simulink model "QUAD_With_IBS_Final"  (R2015a)
settings: Solver=ode45  StartTime=0.0  StopTime=10.0  RelTol=1e-3
libraries: simulink x10, commnoisgen2 x6
settings Model: Creator=Oussama  LastModifiedBy=Oussama

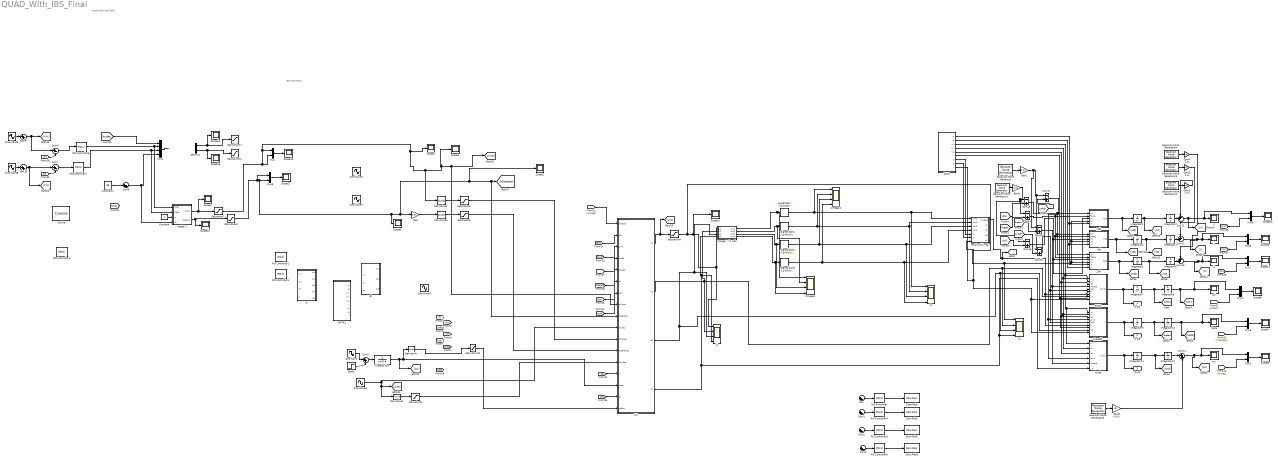
== system QUAD_With_IBS_Final ==
  note: IBS CONTROL
  note: used to extract data
  Bi : MATLAB Function  TreatAsAtomicUnit=on
  Constant : Constant
  Constant1 : Constant  Value=25
  Cosine : simulink/Lookup Tables/Cosine  Formula=cos(2*pi*u)  NumDataPoints=(2^5)+1  OutputWordLength=16  InternalRulePriority=Speed
  DATA : MATLAB Function  TreatAsAtomicUnit=on
  DATA1 : MATLAB Function  TreatAsAtomicUnit=on
  Demux1 : Demux  Outputs=2
  Derivative{,1..3} (4 alike) : Derivative
  Gain : Gain  Gain=0.01
  Gain1 : Gain  Gain=0.01
  Gain2 : Gain  Gain=0.03
  Gain3 : Gain  Gain=0.03
  Gain4 : Gain  Gain=0.03
  Gain5 : Gain  Gain=0.01
  Gain6 : Gain  Gain=0.0001
  Gaussian Noise Generator : commnoisgen2/Gaussian Noise Generator  m=0  d=1  s=41  Ts=0.02  frameBased=off  sampPerFrame=1  orient=off  outDataType=double
  Gaussian Noise Generator1 : commnoisgen2/Gaussian Noise Generator  m=0  d=1  s=41  Ts=0.02  frameBased=off  sampPerFrame=1  orient=off  outDataType=double
  Gaussian Noise Generator2 : commnoisgen2/Gaussian Noise Generator  m=0.3  d=1  s=41  Ts=5  frameBased=off  sampPerFrame=1  orient=off  outDataType=double
  Gaussian Noise Generator3 : commnoisgen2/Gaussian Noise Generator  m=0.3  d=1  s=41  Ts=12  frameBased=off  sampPerFrame=1  orient=off  outDataType=double
  Gaussian Noise Generator4 : commnoisgen2/Gaussian Noise Generator  m=0.3  d=1  s=41  Ts=7  frameBased=off  sampPerFrame=1  orient=off  outDataType=double
  Gaussian Noise Generator5 : commnoisgen2/Gaussian Noise Generator  m=0  d=1  s=41  Ts=0.02  frameBased=off  sampPerFrame=1  orient=off  outDataType=double
  Integrator{1..12} (12 alike) : Integrator
  Mux{,2..8} (8 alike) : Mux  Inputs=2
  Mux1 : Mux
  Omega i ^2  calc : MATLAB Function  TreatAsAtomicUnit=on
  Omegas : Scope  NumInputPorts=4
      settings: YMin=-5~-5~-5~-5  YMax=5~5~5~5  SaveName=ScopeData3
  PID Controller{,4..6} (4 alike) : simulink/Continuous/PID Controller  Controller=PID  TimeDomain=Continuous-time  SampleTime=-1  IntegratorMethod=Forward Euler  FilterMethod=Forward Euler  Form=Parallel  UseFilter=on  ControllerParametersSource=internal  P=0.696663945518539  I=69.3627675374527  D=0.000480635781112464  N=569.937710840054  InitialConditionSource=internal  InitialConditionForIntegrator=0  InitialConditionForFilter=0  ExternalReset=none  LimitOutput=off  UpperSaturationLimit=+12  LowerSaturationLimit=-12  LinearizeAsGain=on  AntiWindupMode=clamping  Kb=1  TrackingMode=off  Kt=1  PParamMin=[]  PParamMax=[]  IParamMin=[]  IParamMax=[]  DParamMin=[]  DParamMax=[]  NParamMin=[]  NParamMax=[]  KbParamMin=[]  KbParamMax=[]  KtParamMin=[]  KtParamMax=[]  POutMin=[]  POutMax=[]  IOutMin=[]  IOutMax=[]  DOutMin=[]  DOutMax=[]  NOutMin=[]  NOutMax=[]  KbOutMin=[]  KbOutMax=[]  KtOutMin=[]  KtOutMax=[]  IntegratorOutMin=[]  IntegratorOutMax=[]  FilterOutMin=[]  FilterOutMax=[]  SumOutMin=[]  SumOutMax=[]  SumI1OutMin=[]  SumI1OutMax=[]  SumI2OutMin=[]  SumI2OutMax=[]  SumI3OutMin=[]  SumI3OutMax=[]  SumDOutMin=[]  SumDOutMax=[]  SaturationOutMin=[]  SaturationOutMax=[]  IntegratorContinuousStateAttributes=''  IntegratorStateMustResolveToSignalObject=off  IntegratorRTWStateStorageClass=Auto  FilterContinuousStateAttributes=''  FilterStateMustResolveToSignalObject=off  FilterRTWStateStorageClass=Auto  DifferentiatorICPrevScaledInput=0  DifferentiatorOutMin=[]  DifferentiatorOutMax=[]
  PID Controller1 : simulink/Continuous/PID Controller  Controller=PID  TimeDomain=Continuous-time  SampleTime=-1  IntegratorMethod=Forward Euler  FilterMethod=Forward Euler  Form=Parallel  UseFilter=on  ControllerParametersSource=internal  P=0.8  I=0.4  D=2  N=100  InitialConditionSource=internal  InitialConditionForIntegrator=0  InitialConditionForFilter=0  ExternalReset=none  LimitOutput=off  UpperSaturationLimit=inf  LowerSaturationLimit=-inf  LinearizeAsGain=on  AntiWindupMode=none  Kb=1  TrackingMode=off  Kt=1  PParamMin=[]  PParamMax=[]  IParamMin=[]  IParamMax=[]  DParamMin=[]  DParamMax=[]  NParamMin=[]  NParamMax=[]  KbParamMin=[]  KbParamMax=[]  KtParamMin=[]  KtParamMax=[]  POutMin=[]  POutMax=[]  IOutMin=[]  IOutMax=[]  DOutMin=[]  DOutMax=[]  NOutMin=[]  NOutMax=[]  KbOutMin=[]  KbOutMax=[]  KtOutMin=[]  KtOutMax=[]  IntegratorOutMin=[]  IntegratorOutMax=[]  FilterOutMin=[]  FilterOutMax=[]  SumOutMin=[]  SumOutMax=[]  SumI1OutMin=[]  SumI1OutMax=[]  SumI2OutMin=[]  SumI2OutMax=[]  SumI3OutMin=[]  SumI3OutMax=[]  SumDOutMin=[]  SumDOutMax=[]  SaturationOutMin=[]  SaturationOutMax=[]  IntegratorContinuousStateAttributes=''  IntegratorStateMustResolveToSignalObject=off  IntegratorRTWStateStorageClass=Auto  FilterContinuousStateAttributes=''  FilterStateMustResolveToSignalObject=off  FilterRTWStateStorageClass=Auto  DifferentiatorICPrevScaledInput=0  DifferentiatorOutMin=[]  DifferentiatorOutMax=[]
  PID Controller2 : simulink/Continuous/PID Controller  Controller=PID  TimeDomain=Continuous-time  SampleTime=-1  IntegratorMethod=Forward Euler  FilterMethod=Forward Euler  Form=Parallel  UseFilter=on  ControllerParametersSource=internal  P=1.1  I=0.5  D=4  N=100  InitialConditionSource=internal  InitialConditionForIntegrator=0  InitialConditionForFilter=0  ExternalReset=none  LimitOutput=off  UpperSaturationLimit=inf  LowerSaturationLimit=-inf  LinearizeAsGain=on  AntiWindupMode=none  Kb=1  TrackingMode=off  Kt=1  PParamMin=[]  PParamMax=[]  IParamMin=[]  IParamMax=[]  DParamMin=[]  DParamMax=[]  NParamMin=[]  NParamMax=[]  KbParamMin=[]  KbParamMax=[]  KtParamMin=[]  KtParamMax=[]  POutMin=[]  POutMax=[]  IOutMin=[]  IOutMax=[]  DOutMin=[]  DOutMax=[]  NOutMin=[]  NOutMax=[]  KbOutMin=[]  KbOutMax=[]  KtOutMin=[]  KtOutMax=[]  IntegratorOutMin=[]  IntegratorOutMax=[]  FilterOutMin=[]  FilterOutMax=[]  SumOutMin=[]  SumOutMax=[]  SumI1OutMin=[]  SumI1OutMax=[]  SumI2OutMin=[]  SumI2OutMax=[]  SumI3OutMin=[]  SumI3OutMax=[]  SumDOutMin=[]  SumDOutMax=[]  SaturationOutMin=[]  SaturationOutMax=[]  IntegratorContinuousStateAttributes=''  IntegratorStateMustResolveToSignalObject=off  IntegratorRTWStateStorageClass=Auto  FilterContinuousStateAttributes=''  FilterStateMustResolveToSignalObject=off  FilterRTWStateStorageClass=Auto  DifferentiatorICPrevScaledInput=0  DifferentiatorOutMin=[]  DifferentiatorOutMax=[]
  PID Controller3 : simulink/Continuous/PID Controller  Controller=PID  TimeDomain=Continuous-time  SampleTime=-1  IntegratorMethod=Forward Euler  FilterMethod=Forward Euler  Form=Parallel  UseFilter=on  ControllerParametersSource=internal  P=3  I=0.5  D=0.9  N=100  InitialConditionSource=internal  InitialConditionForIntegrator=0  InitialConditionForFilter=0  ExternalReset=none  LimitOutput=off  UpperSaturationLimit=inf  LowerSaturationLimit=-inf  LinearizeAsGain=on  AntiWindupMode=none  Kb=1  TrackingMode=off  Kt=1  PParamMin=[]  PParamMax=[]  IParamMin=[]  IParamMax=[]  DParamMin=[]  DParamMax=[]  NParamMin=[]  NParamMax=[]  KbParamMin=[]  KbParamMax=[]  KtParamMin=[]  KtParamMax=[]  POutMin=[]  POutMax=[]  IOutMin=[]  IOutMax=[]  DOutMin=[]  DOutMax=[]  NOutMin=[]  NOutMax=[]  KbOutMin=[]  KbOutMax=[]  KtOutMin=[]  KtOutMax=[]  IntegratorOutMin=[]  IntegratorOutMax=[]  FilterOutMin=[]  FilterOutMax=[]  SumOutMin=[]  SumOutMax=[]  SumI1OutMin=[]  SumI1OutMax=[]  SumI2OutMin=[]  SumI2OutMax=[]  SumI3OutMin=[]  SumI3OutMax=[]  SumDOutMin=[]  SumDOutMax=[]  SaturationOutMin=[]  SaturationOutMax=[]  IntegratorContinuousStateAttributes=''  IntegratorStateMustResolveToSignalObject=off  IntegratorRTWStateStorageClass=Auto  FilterContinuousStateAttributes=''  FilterStateMustResolveToSignalObject=off  FilterRTWStateStorageClass=Auto  DifferentiatorICPrevScaledInput=0  DifferentiatorOutMin=[]  DifferentiatorOutMax=[]
  PID Controller7 : simulink/Continuous/PID Controller  Controller=PID  TimeDomain=Continuous-time  SampleTime=-1  IntegratorMethod=Forward Euler  FilterMethod=Forward Euler  Form=Parallel  UseFilter=on  ControllerParametersSource=internal  P=1.9  I=2.5  D=10  N=100  InitialConditionSource=internal  InitialConditionForIntegrator=0  InitialConditionForFilter=0  ExternalReset=none  LimitOutput=off  UpperSaturationLimit=inf  LowerSaturationLimit=-inf  LinearizeAsGain=on  AntiWindupMode=none  Kb=1  TrackingMode=off  Kt=1  PParamMin=[]  PParamMax=[]  IParamMin=[]  IParamMax=[]  DParamMin=[]  DParamMax=[]  NParamMin=[]  NParamMax=[]  KbParamMin=[]  KbParamMax=[]  KtParamMin=[]  KtParamMax=[]  POutMin=[]  POutMax=[]  IOutMin=[]  IOutMax=[]  DOutMin=[]  DOutMax=[]  NOutMin=[]  NOutMax=[]  KbOutMin=[]  KbOutMax=[]  KtOutMin=[]  KtOutMax=[]  IntegratorOutMin=[]  IntegratorOutMax=[]  FilterOutMin=[]  FilterOutMax=[]  SumOutMin=[]  SumOutMax=[]  SumI1OutMin=[]  SumI1OutMax=[]  SumI2OutMin=[]  SumI2OutMax=[]  SumI3OutMin=[]  SumI3OutMax=[]  SumDOutMin=[]  SumDOutMax=[]  SaturationOutMin=[]  SaturationOutMax=[]  IntegratorContinuousStateAttributes=''  IntegratorStateMustResolveToSignalObject=off  IntegratorRTWStateStorageClass=Auto  FilterContinuousStateAttributes=''  FilterStateMustResolveToSignalObject=off  FilterRTWStateStorageClass=Auto  DifferentiatorICPrevScaledInput=0  DifferentiatorOutMin=[]  DifferentiatorOutMax=[]
  PID Controller8 : simulink/Continuous/PID Controller  Controller=PID  TimeDomain=Continuous-time  SampleTime=-1  IntegratorMethod=Forward Euler  FilterMethod=Forward Euler  Form=Parallel  UseFilter=on  ControllerParametersSource=internal  P=2  I=2  D=8  N=100  InitialConditionSource=internal  InitialConditionForIntegrator=0  InitialConditionForFilter=0  ExternalReset=none  LimitOutput=off  UpperSaturationLimit=inf  LowerSaturationLimit=-inf  LinearizeAsGain=on  AntiWindupMode=none  Kb=1  TrackingMode=off  Kt=1  PParamMin=[]  PParamMax=[]  IParamMin=[]  IParamMax=[]  DParamMin=[]  DParamMax=[]  NParamMin=[]  NParamMax=[]  KbParamMin=[]  KbParamMax=[]  KtParamMin=[]  KtParamMax=[]  POutMin=[]  POutMax=[]  IOutMin=[]  IOutMax=[]  DOutMin=[]  DOutMax=[]  NOutMin=[]  NOutMax=[]  KbOutMin=[]  KbOutMax=[]  KtOutMin=[]  KtOutMax=[]  IntegratorOutMin=[]  IntegratorOutMax=[]  FilterOutMin=[]  FilterOutMax=[]  SumOutMin=[]  SumOutMax=[]  SumI1OutMin=[]  SumI1OutMax=[]  SumI2OutMin=[]  SumI2OutMax=[]  SumI3OutMin=[]  SumI3OutMax=[]  SumDOutMin=[]  SumDOutMax=[]  SaturationOutMin=[]  SaturationOutMax=[]  IntegratorContinuousStateAttributes=''  IntegratorStateMustResolveToSignalObject=off  IntegratorRTWStateStorageClass=Auto  FilterContinuousStateAttributes=''  FilterStateMustResolveToSignalObject=off  FilterRTWStateStorageClass=Auto  DifferentiatorICPrevScaledInput=0  DifferentiatorOutMin=[]  DifferentiatorOutMax=[]
  Phidd : MATLAB Function  TreatAsAtomicUnit=on
  Saturation10 : Saturate  UpperLimit=50  LowerLimit=-50
  Saturation11 : Saturate  UpperLimit=0.4  LowerLimit=-0.4
  Saturation12 : Saturate  UpperLimit=0.4  LowerLimit=-0.4
  Saturation4 : Saturate  UpperLimit=25  LowerLimit=1
  Saturation5 : Saturate  UpperLimit=50  LowerLimit=-50
  Saturation6 : Saturate  UpperLimit=50  LowerLimit=-50
  Saturation7 : Saturate  UpperLimit=0.35  LowerLimit=-0.35
  Saturation8 : Saturate  UpperLimit=0.35  LowerLimit=-0.35
  Saturation9 : Saturate  UpperLimit=pi  LowerLimit=-pi
  Scope{1..17} (17 alike) : Scope
      Scope1 settings: TimeRange=10  YMin=-0.504  YMax=-0.491
      Scope10 settings: YMin=4  YMax=5.75  SaveName=xdata
      Scope11 settings: YMin=7.955  YMax=7.9725  SaveName=zdata
      Scope12 settings: YMin=1.5708  YMax=1.5708
      Scope13 settings: TimeRange=10  YMin=-0.504  YMax=-0.491  SaveName=ScopeData17
      Scope14 settings: SaveName=ScopeData18
      Scope15 settings: TimeRange=10  YMin=-1.53062  YMax=-1.53062  SaveName=ScopeData19
      Scope16 settings: YMin=0.399992  YMax=0.400001  SaveName=ScopeData20
      Scope17 settings: TimeRange=10  YMin=-0.2  YMax=-0.185  SaveName=ScopeData21
      Scope2 settings: SaveName=ScopeData8
      Scope3 settings: SaveName=ScopeData9
      Scope4 settings: TimeRange=10  YMin=-0.504  YMax=-0.491  SaveName=ScopeData10
      Scope5 settings: YMin=1.49226  YMax=1.64934  SaveName=ScopeData11
      Scope6 settings: YMin=-0.125  YMax=0.125  SaveName=phi_ang
      Scope7 settings: YMin=-0.525  YMax=-0.275  SaveName=theta_ang
      Scope8 settings: YMin=-0.002  YMax=0  SaveName=ksi_ang
      Scope9 settings: YMin=-15  YMax=7.5  SaveName=ydata
  Signed Sqrt{,1..3} (4 alike) : Sqrt  Operator=signedSqrt  SaturateOnIntegerOverflow=on
  Sine Wave : Sin  Amplitude=0  Frequency=0.5  SampleTime=0
  Sine Wave2 : Sin  Amplitude=0.3  Frequency=0.6  SampleTime=0
  Sine Wave4 : Sin  Amplitude=0.2  Frequency=0.3  SampleTime=0
  Sine Wave5 : Sin  Amplitude=0  Frequency=0.3  SampleTime=0
  Sine Wave7 : Sin  Amplitude=0.3  Frequency=0.6  SampleTime=0
  Sine Wave8 : Sin  Amplitude=10  Frequency=4*0.06  SampleTime=0
  Sine Wave9 : Sin  Amplitude=5  Frequency=5*0.06  Phase=3.14/2  SampleTime=0
  Step1 : Step  After=5  SampleTime=0
  Sum{,1..3,7,9} (6 alike) : Sum  Inputs=|+-
  Sum{5..6,8,10,14} (5 alike) : Sum  Inputs=|++
  Sum11 : Sum  Inputs=++|
  Sum12 : Sum  Inputs=++|
  Sum13 : Sum  Inputs=++|
  Sum{4,15..19} (6 alike) : Sum  Inputs=-+
  Transfer Fcn : TransferFcn  Denominator=[1 0.4]
  Ui : Scope  NumInputPorts=4
      settings: YMin=-5~-5~-5~-5  YMax=5~5~5~5  SaveName=ScopeData15
  Uiii : MATLAB Function  TreatAsAtomicUnit=on
  X : Scope
      settings: YMin=3.81  YMax=3.95  SaveName=ScopeData6
  X1 : Scope  NumInputPorts=4
      settings: YMin=-5~-5~-5~-5  YMax=5~5~5~5  SaveName=ScopeData16
  X2 : Scope  NumInputPorts=4
      settings: YMin=-5~-5~-5~-5  YMax=5~5~5~5  SaveName=ScopeData7
  Xdd : MATLAB Function  TreatAsAtomicUnit=on
  Y : Scope
      settings: YMin=-0.01095  YMax=-0.0103  SaveName=ScopeData5
  Ydd : MATLAB Function  TreatAsAtomicUnit=on
  "Z " : Scope
      settings: YMin=7.615  YMax=7.6215  SaveName=ScopeData2
  Zdd : MATLAB Function  TreatAsAtomicUnit=on
  Zero-Pole{,1..3} (4 alike) : ZeroPole  Zeros=[]  Poles=[-22.5]  Gain=[509]
  "ai " : MATLAB Function  TreatAsAtomicUnit=on
  angles 1 : MATLAB Function  TreatAsAtomicUnit=on
  ksi : Scope
      settings: SaveName=ksiangle
  ksidd : MATLAB Function  TreatAsAtomicUnit=on
  omegas2 : Scope  NumInputPorts=4
      settings: YMin=-5~-5~-5~-5  YMax=5~5~5~5  SaveName=ScopeData4
  phi : Scope
      settings: SaveName=phiangle
  recalc of Ui real : MATLAB Function  TreatAsAtomicUnit=on
  theta : Scope
      settings: SaveName=thetaangle
  thetadd : MATLAB Function  TreatAsAtomicUnit=on
  Out2 : Outport
  Out3 : Outport  Port=2
  Out4 : Outport  Port=3
  wires:
  Xdd/1(Xdd) -> [Xdd], Integrator1/1
  Ydd/1(Ydd) -> [Ydd], Integrator3/1
  Zdd/1(Zdd) -> [zdd], Integrator5/1
  Phidd/1(phidd) -> Out2/1, Integrator7/1
  Integrator7/1 -> [phid], Integrator8/1
  thetadd/1(thetadd) -> Out3/1, Integrator9/1
  Integrator9/1 -> [thetad], Integrator10/1
  ksidd/1(ksidd) -> Out4/1, Integrator11/1
  Integrator11/1 -> [ksid], Integrator12/1
  Integrator8/1 -> Mux2/1, phi/1, [phi]
  DATA/1(m) -> Zdd/5(m), Ydd/5(m), Xdd/5(m)
  DATA/2(g) -> Zdd/6(g)
  DATA/3(Ixx) -> ksidd/1(Ixx), thetadd/1(Ixx), Phidd/1(Ixx)
  DATA/4(Iyy) -> Phidd/2(Iyy), ksidd/2(Iyy), thetadd/2(Iyy)
  DATA/5(Izz) -> thetadd/3(Izz), ksidd/3(Izz), Phidd/3(Izz)
  DATA/6(J) -> thetadd/7(J), Phidd/7(J)
  Sum15/1 -> Zdd/1(phi), Ydd/1(phi), Xdd/1(phi)
  Sum4/1 -> Zdd/2(theta), Ydd/2(theta), Xdd/2(theta)
  Sum16/1 -> Xdd/3(ksi), Zdd/3(ksi), Ydd/3(ksi)
  Sum18/1 -> Phidd/4(thetad), ksidd/5(thetad)
  Sum19/1 -> Phidd/5(ksid), thetadd/5(ksid)
  Sum17/1 -> ksidd/4(phid), thetadd/4(phid)
  recalc of Ui real/1(omega) -> [omega], thetadd/6(omega), Phidd/6(omega)
  DATA/7(b) -> recalc of Ui real/5(b)
  DATA/8(d) -> recalc of Ui real/6(d)
  Uiii/4(U4) -> ksidd/6(u4), X2/4, Ui/4, Omega i ^2  calc/4(u4)
  Uiii/3(U3) -> X2/3, thetadd/8(u3), Ui/3, Omega i ^2  calc/3(u3)
  Uiii/2(U2) -> X2/2, Phidd/8(u2), Omega i ^2  calc/2(u2), Ui/2
  Omega i ^2  calc/1(om1) -> Omegas/1, Signed Sqrt/1
  Omega i ^2  calc/2(om2) -> Omegas/2, Signed Sqrt1/1
  Omega i ^2  calc/3(om3) -> Omegas/3, Signed Sqrt2/1
  Omega i ^2  calc/4(om4) -> Omegas/4, Signed Sqrt3/1
  Gain5/1 -> Sum16/1, Sum4/1, Sum15/1
  [phi] -> Sum15/2
  [theta] -> Sum4/2
  [ksi] -> Sum16/2
  Gain1/1 -> Sum18/1, Sum19/1, Sum17/1
  [phid] -> Sum17/2
  [thetad] -> Sum18/2
  [ksid] -> Sum19/2
  Saturation4/1 -> X2/1, Zdd/4(u1), Ydd/4(u1), Xdd/4(u1), Scope14/1, Ui/1, Omega i ^2  calc/1(u1)
  Integrator5/1 -> [zd], Integrator6/1
  Integrator3/1 -> [Yd], Integrator4/1
  Integrator1/1 -> [Xd], Integrator2/1
  DATA/9(l) -> Phidd/9(l), thetadd/9(l), recalc of Ui real/7(l)
  [phides] -> Mux2/2
  Mux2/1 -> Scope6/1
  Integrator10/1 -> [theta], Mux3/1, theta/1
  [thetades] -> Mux3/2
  Mux3/1 -> Scope7/1
  Sum14/1 -> [ksi], Mux4/1, ksi/1
  [ksides] -> Mux4/2
  Mux4/1 -> Scope8/1
  Sum12/1 -> [Y], Mux5/1, Y/1
  [YYY] -> Mux5/2
  Mux5/1 -> Scope9/1
  Sum11/1 -> [X], Mux6/1, X/1
  [XXX] -> Mux6/2
  Mux6/1 -> Scope10/1
  Sum13/1 -> Mux7/1, "Z "/1, [Z]
  [zzz] -> Mux7/2
  Mux7/1 -> Scope11/1
  Sum5/1 -> Transfer Fcn/1
  Derivative/1 -> Saturation10/1
  Sine Wave5/1 -> Derivative1/1, [ksides], Uiii/10(ksides)
  Derivative1/1 -> Saturation9/1
  [omega] -> Uiii/1(omega)
  Uiii/1(U1) -> [U11], Saturation4/1
  Step1/1 -> Sum5/2
  Sine Wave/1 -> Sum5/1
  Derivative2/1 -> Saturation5/1
  Derivative3/1 -> Saturation6/1
  ? -> Sum/2
  Sum/1 -> PID Controller/1
  PID Controller/1 -> Zero-Pole/1
  ? -> Sum1/2
  Sum1/1 -> PID Controller4/1
  PID Controller4/1 -> Zero-Pole1/1
  ? -> Sum2/2
  Sum2/1 -> PID Controller5/1
  PID Controller5/1 -> Zero-Pole2/1
  ? -> Sum3/2
  Sum3/1 -> PID Controller6/1
  PID Controller6/1 -> Zero-Pole3/1
  Signed Sqrt/1 -> X1/1, recalc of Ui real/1(om1), omegas2/1
  Signed Sqrt1/1 -> X1/2, recalc of Ui real/2(om2), omegas2/2
  Signed Sqrt2/1 -> X1/3, recalc of Ui real/3(om3), omegas2/3
  Signed Sqrt3/1 -> X1/4, recalc of Ui real/4(om4), omegas2/4
  [phi] -> Uiii/2(phi)
  [theta] -> Uiii/4(theta)
  [thetad] -> Uiii/5(thetad)
  [ksi] -> Uiii/6(ksi)
  [ksid] -> Uiii/7(ksid)
  [phid] -> Uiii/3(phid)
  Saturation9/1 -> Uiii/13(ksiddes)
  Saturation7/1 -> Mux/2, Derivative2/1, Uiii/8(phides), [phides], Scope3/1, Scope4/1, Mux/1
  Saturation8/1 -> Mux8/2, Scope5/1, Gain/1, Scope2/1, Uiii/9(thetades), [thetades], Mux8/1
  Saturation5/1 -> Uiii/11(phiddes)
  Saturation6/1 -> Uiii/12(thetaddes)
  [Z] -> Uiii/14(z)
  [zd] -> Uiii/16(zd)
  Saturation10/1 -> Uiii/17(zddes)
  Mux1/1 -> ?
  Demux1/1 -> Scope15/1, Saturation11/1
  Demux1/2 -> Saturation12/1, Scope16/1
  ? -> Demux1/1
  [ksides] -> Mux1/1
  Sum6/1 -> Mux1/4, angles 1/4(U1)
  Constant/1 -> angles 1/3(m)
  angles 1/1(phitrk) -> Saturation7/1, Scope1/1
  angles 1/2(thetatrk) -> Scope12/1, Saturation8/1
  Mux/1 -> Scope13/1
  Mux8/1 -> Scope17/1
  Sum8/1 -> Sum9/1, [XXX]
  Sum10/1 -> [YYY], Sum7/1
  Sine Wave8/1 -> Sum10/1
  Sine Wave9/1 -> Sum8/1
  Sum9/1 -> PID Controller8/1
  Sum7/1 -> PID Controller7/1
  [X] -> Sum9/2
  [Y] -> Sum7/2
  Constant1/1 -> Sum6/1
  PID Controller7/1 -> angles 1/2(Ydes), Mux1/3
  PID Controller8/1 -> angles 1/1(Xdes), Mux1/2
  Gain/1 -> Derivative3/1
  Transfer Fcn/1 -> [zzz], Uiii/15(zdes), Derivative/1
  Gaussian Noise Generator2/1 -> Gain2/1
  Gain2/1 -> Sum11/1
  Gaussian Noise Generator3/1 -> Gain3/1
  Gain3/1 -> Sum12/1
  Gaussian Noise Generator4/1 -> Gain4/1
  Gain4/1 -> Sum13/1
  Gaussian Noise Generator/1 -> Gain1/1
  Gaussian Noise Generator1/1 -> Gain5/1
  Integrator2/1 -> Sum11/2
  Integrator4/1 -> Sum12/2
  Integrator6/1 -> Sum13/2
  Gaussian Noise Generator5/1 -> Gain6/1
  Integrator12/1 -> Sum14/1
  Gain6/1 -> Sum14/2

== matlab function QUAD_With_IBS_Final/Ydd ==
  data: phi input; Ydd output; theta input; ksi input; u1 input; m input
function Ydd = fcn(phi,theta, ksi,u1,m)
m=1;

Ydd=(-cos(ksi)*sin(phi)+sin(ksi)*sin(theta)*cos(phi))*u1/m;

== matlab function QUAD_With_IBS_Final/Zdd ==
  data: phi input; Zdd output; theta input; ksi input; u1 input; m input; g input
function Zdd = fcn(phi,theta, ksi,u1,m,g)
m=1;
g=9.81;

Zdd=-g+(cos(theta)*cos(phi))*u1/m;

== matlab function QUAD_With_IBS_Final/DATA ==
  data: m output; g output; Ixx output; Iyy output; Izz output; J output; b output; d output; l output
function [m,g,Ixx,Iyy,Izz,J,b,d,l] = fcn
m=1;
g=9.81;

Ixx=1*0.008;
Iyy=1*0.008;
Izz=1*0.015;
b=0.0001;
d=0.000001;
l=0.25;
J=0.0001;

== matlab function QUAD_With_IBS_Final/Phidd ==
  data: Ixx input; Iyy input; phidd output; Izz input; thetad input; ksid input; omega input; J input; u2 input; l input
function phidd = fcn(Ixx,Iyy,Izz,thetad, ksid,omega,J,u2,l)


phidd=1/Ixx*((Iyy-Izz)*thetad*ksid-J*thetad*omega+l*u2);

== matlab function QUAD_With_IBS_Final/thetadd ==
  data: Ixx input; Iyy input; thetadd output; Izz input; phid input; ksid input; omega input; J input; u3 input; l input
function thetadd = fcn(Ixx,Iyy,Izz,phid, ksid,omega,J,u3,l)


thetadd=1/Iyy*((Izz-Ixx)*phid*ksid+J*phid*omega+l*u3);

== matlab function QUAD_With_IBS_Final/ksidd ==
  data: Ixx input; Iyy input; ksidd output; Izz input; phid input; thetad input; u4 input
function ksidd = fcn(Ixx,Iyy,Izz,phid, thetad,u4)


ksidd=1/Izz*((Ixx-Iyy)*phid*thetad+u4);

== matlab function QUAD_With_IBS_Final/Omega i ^2  calc ==
  data: u1 input; om1 output; u2 input; u3 input; u4 input; om2 output; om3 output; om4 output
function [om1,om2,om3,om4] = fcn(u1,u2,u3,u4)
%#codegen
b=0.0001;
d=0.000001;
l=0.25;
A=[ 1/(4*b),0, -1/(2*b*l), -1/(4*d);1/(4*b), -1/(2*b*l),0,  1/(4*d); 1/(4*b),  0,  1/(2*b*l), -1/(4*d);1/(4*b),1/(2*b*l), 0,  1/(4*d)];
B=A*[u1;u2;u3;u4];
%[om1;om2;om3;om4]
om1= B(1);
om2=B(2);
om3=B(3);
om4=B(4);

== matlab function QUAD_With_IBS_Final/ai  ==
  data: Ixx input; a1 output; Iyy input; Izz input; a2 output; a3 output; a4 output; a5 output; Jr input
function [a1,a2,a3,a4,a5] = fcn(Ixx,Iyy,Izz,Jr)
a1=(Iyy-Izz)/Ixx;
a2=-Jr/Ixx;
a3=(Izz-Ixx)/Iyy;
a4=Jr/Iyy;
a5=(Ixx-Iyy)/Izz;

== matlab function QUAD_With_IBS_Final/Xdd ==
  data: phi input; Xdd output; theta input; ksi input; u1 input; m input
function Xdd = fcn(phi,theta, ksi,u1,m)


Xdd=(sin(ksi)*sin(phi)+cos(ksi)*sin(theta)*cos(phi))*u1/m;

== matlab function QUAD_With_IBS_Final/recalc of Ui real ==
  data: om1 input; omega output; om2 input; om3 input; om4 input; b input; d input; l input; u1 output; u2 output; u3 output; u4 output
function [omega, u1,u2,u3,u4] = fcn(om1,om2,om3,om4,b,d,l)

l=l;
omega=-om1+om2-om3+om4;
u1=b*(om1^2+om2^2+om3^2+om4^2);
u2=b*(om4^2-om2^2);
u3=b*(om3^2-om1^2);
u4=d*(om4^2+om2^2-om1^2-om3^2);

== matlab function QUAD_With_IBS_Final/Bi ==
  data: l input; Ixx input; b1 output; Iyy input; Izz input; b2 output; b3 output
function [b1,b2,b3] = fcn(l,Ixx,Iyy,Izz)

b1= l/Ixx;
b2= l/Iyy;
b3= l/Izz;

== matlab function QUAD_With_IBS_Final/angles 1 ==
  data: Xdes input; phitrk output; Ydes input; m input; U1 input; thetatrk output
function [phitrk,thetatrk]  = fcn(Xdes,Ydes, m,U1)
%#codegen
if U1<=5
    phitrk=0;
else
    if (abs(Ydes*m/U1) >= 0.3)
        phitrk= -sign(Ydes*m/U1)*pi/10;
    else
    phitrk=-asin(Ydes*m/U1);
    end
end
%%%%%%%%%%%%%%%%%%
if U1<=5
    thetatrk=0;
elseif (abs( Xdes*m/(U1*cos(phitrk)) ) >= 0.3 )
        thetatrk = sign( Xdes*m/(U1*cos(phitrk)) )*pi/10 ;
    else
    thetatrk=asin(Xdes*m/(U1*cos(phitrk)) );
end

    
%%%%%%%%%%%%
if phitrk > pi/3
    phitrk=pi/3;
end
if phitrk < -pi/3
    phitrk=-pi/3;
end
%%%%%%%%%%%%%%%
if thetatrk > pi/3
    thetatrk=pi/3;
end
if thetatrk < -pi/3
    thetatrk=-pi/3;
end

== matlab function QUAD_With_IBS_Final/DATA1 ==
  data: m output; g output; Ixx output; Iyy output; Izz output; J output; b output; d output; l output
function [m,g,Ixx,Iyy,Izz,J,b,d,l] = fcn
m=1;
g=9.81;

Ixx=1*0.008;
Iyy=1*0.008;
Izz=1*0.015;
b=0.0001;
d=0.000001;
l=0.25;
J=0.0001;

== matlab function QUAD_With_IBS_Final/Uiii ==
  data: omega input; phi input; phid input; theta input; thetad input; ksi input; ksid input; phides input; U1 output; U2 output; thetades input; ksides input; phiddes input; thetaddes input; ksiddes input; U3 output; U4 output; z input; zdes input; zd input; zddes input
function [U1,U2,U3,U4] = fcn(omega,phi,phid,theta,thetad,ksi,ksid,phides,thetades,ksides,phiddes,thetaddes,ksiddes,z,zdes,zd,zddes)
%%%%%%%%%%%%%%%%%%%%%%%%%%%%%%%%%%%%%%%%%%%%%%%%%%%%%%%%%%%%%
%%%%%%%%%%%%%%%%%%%%%%%%%%%%%%%%%%%%%%%%%%%%%%%%%%%%%%%%%%%%%

m=1;
g=9.81;

Ixx=1*0.008;
Iyy=1*0.008;
Izz=1*0.015;
b=0.0001;
d=0.000001;
l=0.25;
J=0.0001;
%%%%%%%%%%%%%%%%%%%%%%%%%%%%%%%%%%%%%%%%%%%%%%%%%%%%%%%%%%%%%
%%%%%%%%%%%%%%%%%%%%%%%%%%%%%%%%%%%%%%%%%%%%%%%%%%%%%%%%%%%%%

a1=(Iyy-Izz)/Ixx;
a2=-J/Ixx;
a3=(Izz-Ixx)/Iyy;
a4=J/Iyy;
a5=(Ixx-Iyy)/Izz;
%%%%%%%%%%%%%%%%%%%%%%%%%%%%%%%%%%%%%%%%%%%%%%%%%%%%%%%%%%%%%
%%%%%%%%%%%%%%%%%%%%%%%%%%%%%%%%%%%%%%%%%%%%%%%%%%%%%%%%%%%%%
b1= l/Ixx;
b2= l/Iyy;
b3= l/Izz;

%%%%%%%%%%%%%%%%%%%%%%%%%%%%%%%%%%%%%%%%%%%%%%%%%%%%%%%%%%%%%
%%%%%%%%%%%%%%%%%%%%%%%%%%%%%%%%%%%%%%%%%%%%%%%%%%%%%%%%%%%%%

k1=5.3;
k2=2.9;
k3=4.4;
k4=3.7;
k5=3.5;
k6=2.6;
k7=4.7;
k8=2.8;

% k7=1.7;
% k8=0.8;
%%%%%%%%%%%%%%%%%%%%%%%%%%%%%%%%%%%%%%%%%%%%%%%%%%%%%%%%%%%%%
%%%%%%%%%%%%%%%%%%%%%%%%%%%%%%%%%%%%%%%%%%%%%%%%%%%%%%%%%%%%%

z1=phides-phi;
z2=phid-phiddes-k1*z1;

z3=thetades-theta;
z4=thetad-thetaddes-k3*z3;

z5=ksides-ksi;
z6=ksid-ksiddes-k5*z5;

z7=zdes-z;
z8=zd-zddes-k7*z7;
%%%%%%%%%%%%%%%%%%%%%%%%%%%%%%%%%%%%%%%%%%%%%%%%%%%%%%%%%%%%%
%%%%%%%%%%%%%%%%%%%%%%%%%%%%%%%%%%%%%%%%%%%%%%%%%%%%%%%%%%%%%

U1=  (m/(cos(phi)*cos(theta)))*(z7+g-k7*(z8+k7*z7)-k8*z8) ;

U2= 1/b1*(z1-a1*thetad*ksid-a2*thetad*omega-k1*(z2+k1*z1)-k2*z2)  ; 

U3=  1/b2*(z3-a3*phid *ksid-a4*phid  *omega-k3*(z4+k3*z3)-k4*z4) ;

U4=   1/b3*(z5-a5*phid*thetad-k5*(z6+k5*z5)-k6*z6);
